simulink model "multimanchester"  (Simulink 5.1)
settings: Solver=FixedStepDiscrete  SolverMode=SingleTasking  StartTime=0.0  StopTime=50000.0  RelTol=1e-3
undefined symbols (not defined in the file or in its folder): sigbuilder_block
libraries: fixpt_lib_4 x5, dspsigops x5, modelsimlib x3, simulink x2, dspsrcs4 x1
settings Model: Creator=bogilvie  LastModifiedBy=bogilvie  BlockReductionOpt=off  BooleanDataType=on  ProdHWDeviceType=Microprocessor

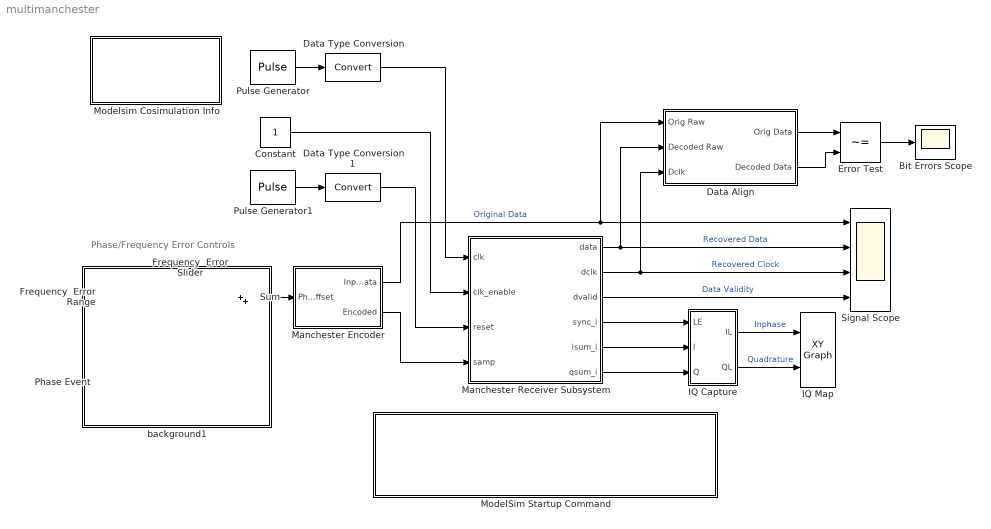
== system multimanchester ==
  note: Phase/Frequency Error Controls
  Bit Errors Scope : Scope
      settings: TimeRange=3000  YMin=-1  YMax=1
  Constant : Constant  ShowAdditionalParam=on  OutDataTypeMode=boolean  SampleTime=5
  Data Align : Subsystem
  Data Type Conversion : DataTypeConversion  DataType=boolean  SaturateOnIntegerOverflow=on
  Data Type Conversion1 : DataTypeConversion  DataType=boolean  SaturateOnIntegerOverflow=on
  Error Test : RelationalOperator  Operator=~=  ShowAdditionalParam=on  LogicOutDataTypeMode=Boolean  ZeroCross=off
  Frequency  Error Range : dspsrcs4/DSP Constant  Value=1/128  SampleMode=Discrete  discreteOutput=Sample-based  continuousOutput=Sample-based  sampTime=10  framePeriod=2  dataType=Inherit from 'Constant value'  wordLen=16  udDataType=sfix(16)  fracBitsMode=Best precision  numFracBits=15  InterpretAs1D=-inf  Ts=-inf  FramebasedOutput=-inf
  Frequency  Error Slider : simulink/Math Operations/Slider Gain  low=-1  gain=0  high=1
  IQ Capture : Subsystem
  IQ Map : simulink/Sinks/XY Graph  xmin=0  xmax=16  ymin=0  ymax=16  st=-1
  Manchester Encoder : Subsystem
  Manchester Receiver Subsystem : Subsystem
  ModelSim Startup Command : Subsystem
      settings: OpenFcn=vsim('tclstart',multimanchestercmds);
      mask Display: disp(['vsim(''tclkstart'',multimanchestercmds)', char(10), '%', 'Double-click here to launch a new ModelSim'])
  Modelsim Cosimulation Info : Subsystem
      settings: OpenFcn=web(fullfile(matlabroot,'toolbox','modelsim','modelsimdemos','html','manchesterreceiverdemo.html'))
      mask Type: VHDL Manchester Receiver Demo Info
      mask Display: disp('VHDL Manchester\nReceiver Simulation\nInformation')
  Phase Event : Subsystem  Tag=STV Subsys  StartFcn=sigbuilder_block('start');  StopFcn=sigbuilder_block('stop');  ClipboardFcn=sigbuilder_block('clipboard');  mask(Sigbuilder block){}
      mask help: Sigbuilder GUI
      mask init:
      | if ~strcmp(get_param(bdroot(gcb),'SimulationStatus'),'stopped') tuvar = sigbuilder_block('maskInit'); end
      settings: CopyFcn=sigbuilder_block('copy');  DeleteFcn=sigbuilder_block('delete');  ModelCloseFcn=sigbuilder_block('modelClose');  PreSaveFcn=sigbuilder_block('preSave');  NameChangeFcn=sigbuilder_block('namechange');  OpenFcn=sigbuilder_block('open',[132.75 331.5 522.75 330 ]);  CloseFcn=sigbuilder_block('close');
      mask Display: plot(0,0,100,100,[10,10,40,40,10],[80,20,20,80,80],[40,10],[50,50], [40,27,10],[65,72,56],[40,25,25,10],[28,28,43,43]);
  Pulse Generator : DiscretePulseGenerator  SampleTime=5
  Pulse Generator1 : DiscretePulseGenerator  Period=10000  PulseWidth=200  SampleTime=5
  Signal Scope : Scope  NumInputPorts=4
      settings: TimeRange=3000  YMin=-1~-1~-1~0.95  YMax=2~2~2~1.05
  Sum : Sum  Inputs=|++  SaturateOnIntegerOverflow=on
  background1 : Subsystem
      mask Display: disp('')
  wires:
  Manchester Encoder/2(Encoded) -> Manchester Receiver Subsystem/4(samp)
  Manchester Receiver Subsystem/3(dvalid) -> Signal Scope/4  "Data Validity"
  Sum/1 -> Manchester Encoder/1(Phase Offset)
  Phase Event/1(Signal 1) -> Sum/2
  Manchester Receiver Subsystem/2(dclk) -> Signal Scope/3, Data Align/3(Dclk)  "Recovered Clock"
  Manchester Encoder/1(Input Data) -> Signal Scope/1, Data Align/1(Orig Raw)  "Original Data"
  Frequency  Error Range/1 -> Frequency  Error Slider/1
  Frequency  Error Slider/1 -> Sum/1
  Manchester Receiver Subsystem/1(data) -> Signal Scope/2, Data Align/2(Decoded Raw)  "Recovered Data"
  Manchester Receiver Subsystem/4(sync_i) -> IQ Capture/1(LE)
  Manchester Receiver Subsystem/6(qsum_i) -> IQ Capture/3(Q)
  Manchester Receiver Subsystem/5(isum_i) -> IQ Capture/2(I)
  Data Align/1(Orig Data) -> Error Test/1
  Data Align/2(Decoded Data) -> Error Test/2
  Error Test/1 -> Bit Errors Scope/1
  IQ Capture/1(IL) -> IQ Map/1  "Inphase"
  IQ Capture/2(QL) -> IQ Map/2  "Quadrature"
  Pulse Generator1/1 -> Data Type Conversion1/1
  Constant/1 -> Manchester Receiver Subsystem/2(clk_enable)
  Pulse Generator/1 -> Data Type Conversion/1
  Data Type Conversion/1 -> Manchester Receiver Subsystem/1("clk ")
  Data Type Conversion1/1 -> Manchester Receiver Subsystem/3(reset)

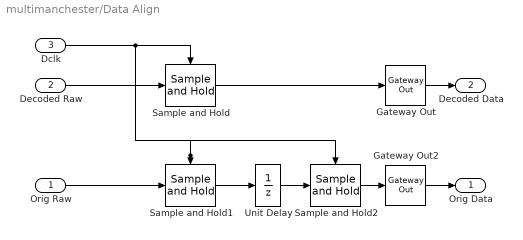
== system multimanchester/Data Align ==
  Orig Raw : Inport
  Decoded Raw : Inport  Port=2
  Dclk : Inport  Port=3
  Gateway Out : fixpt_lib_4/Data Type/Gateway Out  OutRealWorld=Real World Value  OutBuiltInType=double  RndMeth=Nearest  DoSatur=off
  Gateway Out2 : fixpt_lib_4/Data Type/Gateway Out  OutRealWorld=Real World Value  OutBuiltInType=double  RndMeth=Nearest  DoSatur=off
  Sample and Hold : dspsigops/Sample and Hold  trig=Rising edge  initCond=0
  Sample and Hold1 : dspsigops/Sample and Hold  trig=Rising edge  initCond=0
  Sample and Hold2 : dspsigops/Sample and Hold  trig=Rising edge  initCond=0
  Unit Delay : UnitDelay  X0=0.0  SampleTime=-1
  Orig Data : Outport
  Decoded Data : Outport  Port=2
  wires:
  Sample and Hold1/1 -> Unit Delay/1
  Decoded Raw/1 -> Sample and Hold/1
  Orig Raw/1 -> Sample and Hold1/1
  Sample and Hold/1 -> Gateway Out/1
  Unit Delay/1 -> Sample and Hold2/1
  Sample and Hold2/1 -> Gateway Out2/1
  Gateway Out/1 -> Decoded Data/1
  Gateway Out2/1 -> Orig Data/1
  Dclk/1 -> Sample and Hold/Trigger, Sample and Hold1/Trigger, Sample and Hold2/Trigger

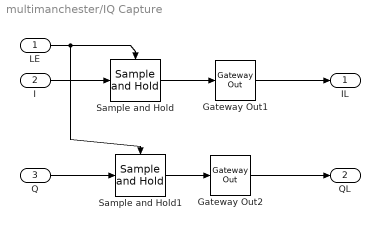
== system multimanchester/IQ Capture ==
  LE : Inport
  I : Inport  Port=2
  Q : Inport  Port=3
  Gateway Out1 : fixpt_lib_4/Data Type/Gateway Out  OutRealWorld=Real World Value  OutBuiltInType=double  RndMeth=Nearest  DoSatur=off
  Gateway Out2 : fixpt_lib_4/Data Type/Gateway Out  OutRealWorld=Real World Value  OutBuiltInType=double  RndMeth=Nearest  DoSatur=off
  Sample and Hold : dspsigops/Sample and Hold  trig=Rising edge  initCond=0
  Sample and Hold1 : dspsigops/Sample and Hold  trig=Rising edge  initCond=0
  IL : Outport
  QL : Outport  Port=2
  wires:
  LE/1 -> Sample and Hold/Trigger, Sample and Hold1/Trigger
  Sample and Hold/1 -> Gateway Out1/1
  Sample and Hold1/1 -> Gateway Out2/1
  Gateway Out1/1 -> IL/1
  Gateway Out2/1 -> QL/1
  I/1 -> Sample and Hold/1
  Q/1 -> Sample and Hold1/1

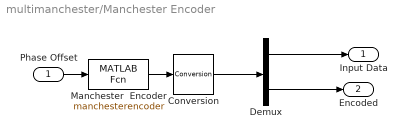
== system multimanchester/Manchester Encoder ==
  Phase Offset : Inport
  Conversion : fixpt_lib_4/Data Type/Conversion  ConvertRealWorld=Real World Value  OutputDataTypeScalingMode=Specify via dialog  OutDataType=ufix(1)  OutScaling=1  DoSatur=off
  Demux : Demux  Outputs=2
  Manchester  Encoder : MATLABFcn  MATLABFcn=manchesterencoder  SampleTime=10
  Input Data : Outport
  Encoded : Outport  Port=2
  wires:
  Manchester  Encoder/1 -> Conversion/1
  Conversion/1 -> Demux/1
  Demux/1 -> Input Data/1
  Phase Offset/1 -> Manchester  Encoder/1
  Demux/2 -> Encoded/1

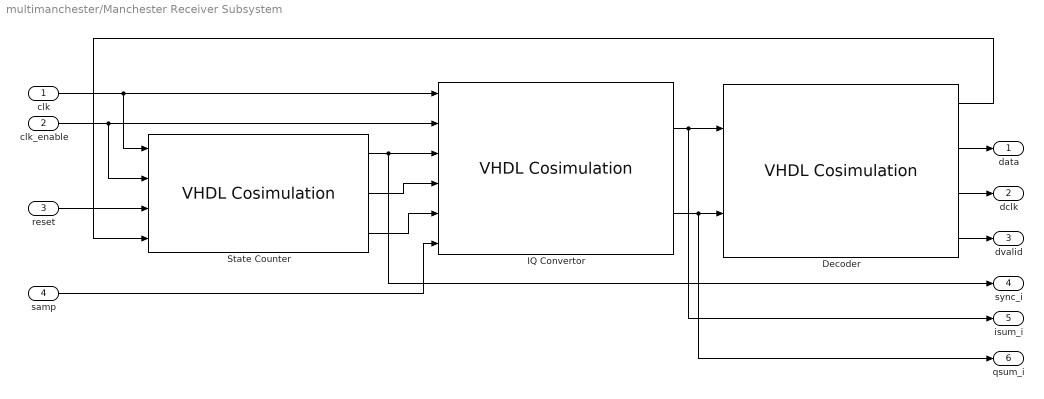
== system multimanchester/Manchester Receiver Subsystem ==
  "clk " : Inport
  clk_enable : Inport  Port=2
  reset : Inport  Port=3
  samp : Inport  Port=4
  Decoder : modelsimlib/VHDL Cosimulation  idxCellArray={'/multimanchester/decoder_isum', 'in', '/multimanchester/decoder_qsum', 'in', '/multimanchester/decoder_adj', 'out', '/multimanchester/data', 'out', '/multimanchester/dclk', 'out', '/multimanchester/dvalid', 'out'}  Tso=-1  tclBefore="echo \"Running Simulink Cosimulation block Decoder.\""  modelSimRunning=on  sharedMemory=on
  IQ Convertor : modelsimlib/VHDL Cosimulation  idxCellArray={'/multimanchester/iqconv_clk', 'in', '/multimanchester/iqconv_enable', 'in', '/multimanchester/iqconv_sync', 'in', '/multimanchester/iqconv_i_wf', 'in', '/multimanchester/iqconv_q_wf', 'in', '/multimanchester/iqconv_samp', 'in', '/multimanchester/iqconv_isum', 'out', '/multimanchester/iqconv_qsum', 'out'}  Tso=-1  tclBefore="echo \"Running Simulink Cosimulation block IQ Convertor.\""  modelSimRunning=on  sharedMemory=on
  State Counter : modelsimlib/VHDL Cosimulation  idxCellArray={'/multimanchester/statecnt_clk', 'in', '/multimanchester/statecnt_enable', 'in', '/multimanchester/statecnt_reset', 'in', '/multimanchester/statecnt_adj', 'in', '/multimanchester/statecnt_sync', 'out', '/multimanchester/statecnt_i_wf', 'out', '/multimanchester/statecnt_q_wf', 'out'}  Tso=-1  tclBefore="echo \"Running Simulink Cosimulation block State Counter.\""  modelSimRunning=on  sharedMemory=on
  data : Outport
  dclk : Outport  Port=2
  dvalid : Outport  Port=3
  sync_i : Outport  Port=4
  isum_i : Outport  Port=5
  qsum_i : Outport  Port=6
  wires:
  State Counter/2 -> IQ Convertor/4
  State Counter/1 -> IQ Convertor/3, sync_i/1
  IQ Convertor/1 -> Decoder/1, isum_i/1
  IQ Convertor/2 -> Decoder/2, qsum_i/1
  Decoder/1 -> State Counter/4
  clk_enable/1 -> IQ Convertor/2, State Counter/2
  State Counter/3 -> IQ Convertor/5
  samp/1 -> IQ Convertor/6
  "clk "/1 -> State Counter/1, IQ Convertor/1
  reset/1 -> State Counter/3
  Decoder/2 -> data/1
  Decoder/3 -> dclk/1
  Decoder/4 -> dvalid/1

== system multimanchester/ModelSim Startup Command ==

== system multimanchester/Modelsim Cosimulation Info ==

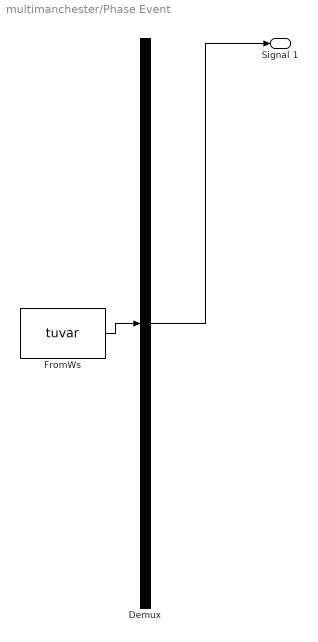
== system multimanchester/Phase Event ==
  Demux : Demux  Tag=STV Demux  Outputs=1
  FromWs : FromWorkspace  Tag=STV FromWs  VariableName=tuvar  SampleTime=10  OutputAfterFinalValue=Holding final value  SigBuilderData=DataTag0
      SigBuilderData=|
      | channels.label = 'Signal 1'
      | channels.allXData = {[0 20020 20020 20570 20570 30000]}
      | channels.allYData = {[0 0 0.0794 0.0794 0 0]}
      | common.afterFinalStr = 'Hold final value'
      | common.sampleTime = 10
      | dataSet.timeRange = [0 30000]
      | dataSet.name = 'Group 1'
  Signal 1 : Outport  Tag=STV Outport
  wires:
  Demux/1 -> Signal 1/1
  FromWs/1 -> Demux/1

== system multimanchester/background1 ==
